simulink model "task_1_2_v01_2017b_compatible"  (R2018a)
settings: Solver=VariableStepAuto  StartTime=0.0  StopTime=1000  RelTol=1e-3
values from neighbouring files (symbols this model uses):
  faultMag = [1 0 0]    [ProblemData.m]
  faultTime = [1e6 1e6 1e6]    [ProblemData.m]
  lambda = 0.5    [ProblemData.m]
  pipeCoeff = [1 1 1]    [ProblemData.m]
  pipeCoeffNom = pipeCoeff * (1 + 0.1 * (rand(1) - 1/2))    [ProblemData.m]
  pipeCross = [5 5 5]*1e-4    [ProblemData.m]
  pipeCrossNom = pipeCross * (1 + 0.1 * (rand(1) - 1/2))    [ProblemData.m]
  pumpConst = [1.5 1.5]*1e-3    [ProblemData.m]
  seed1 = randi([1 100000])    [ProblemData.m]
  seed2 = randi([1 100000])    [ProblemData.m]
  seed3 = randi([1 100000])    [ProblemData.m]
  tankCross = [0.156 0.156 0.156]    [ProblemData.m]
  tankCrossNom = tankCross * (1 + 0.1 * (rand(1) - 1/2))    [ProblemData.m]
  tankInit = [0 2.5 5]    [ProblemData.m]
  tankInitNom = tankInit * (1 + 0.1 * (rand(1) - 1/2))    [ProblemData.m]
  tankMax = [10 10 10]    [ProblemData.m]
  tankMaxNom = tankMax * (1 + 0.1 * (rand(1) - 1/2))    [ProblemData.m]
  tankMin = [0 0 0]    [ProblemData.m]
undefined symbols (not defined in the file or in its folder): DiscIntNeverNeededParam
(part 1 of 2)
settings Model: Creator=riccardoferrar  LastModifiedBy=Casper

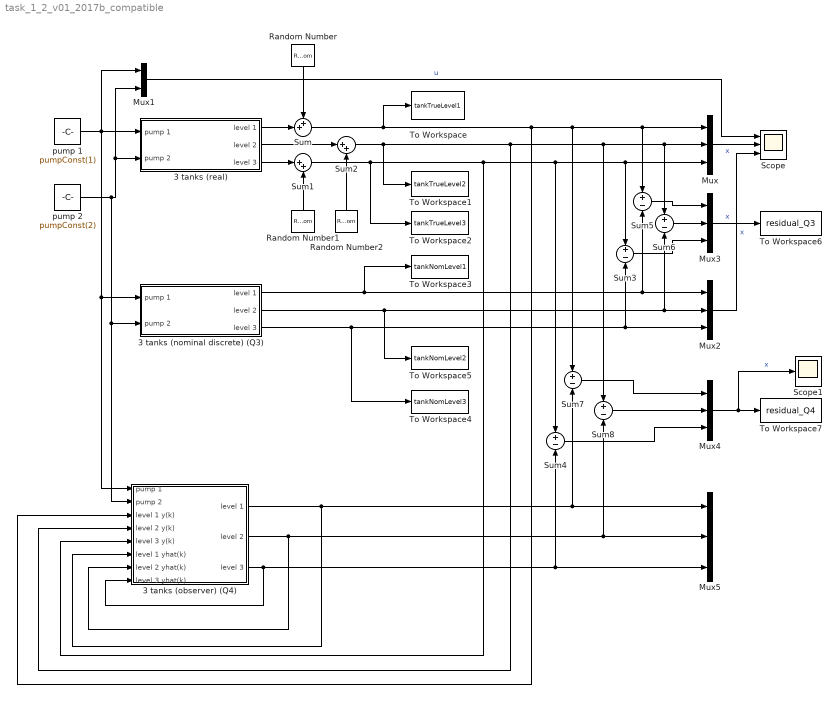
== system task_1_2_v01_2017b_compatible ==
  3 tanks (nominal discrete) (Q3) : Subsystem
  3 tanks (observer) (Q4) : Subsystem
  3 tanks (real) : Subsystem
  Mux{,2..5} (5 alike) : Mux  Inputs=3
  Mux1 : Mux  Inputs=2
  Random Number : RandomNumber  Variance=0.0015  Seed=seed1  SampleTime=0.1
  Random Number1 : RandomNumber  Variance=0.0015  Seed=seed2  SampleTime=0.1
  Random Number2 : RandomNumber  Variance=0.0015  Seed=seed3  SampleTime=0.1
  Scope : Scope  NumInputPorts=3
  Scope1 : Scope
  Sum : Sum  Inputs=++|
  Sum1 : Sum  Inputs=|++
  Sum2 : Sum  Inputs=|++
  Sum{3..8} (6 alike) : Sum  Inputs=+|-
  To Workspace : ToWorkspace  VariableName=tankTrueLevel1  SaveFormat=Timeseries  SampleTime=-1
  To Workspace1 : ToWorkspace  VariableName=tankTrueLevel2  SaveFormat=Timeseries  SampleTime=-1
  To Workspace2 : ToWorkspace  VariableName=tankTrueLevel3  SaveFormat=Timeseries  SampleTime=-1
  To Workspace3 : ToWorkspace  VariableName=tankNomLevel1  SaveFormat=Timeseries  SampleTime=-1
  To Workspace4 : ToWorkspace  VariableName=tankNomLevel3  SaveFormat=Timeseries  SampleTime=-1
  To Workspace5 : ToWorkspace  VariableName=tankNomLevel2  SaveFormat=Timeseries  SampleTime=-1
  To Workspace6 : ToWorkspace  VariableName=residual_Q3  SaveFormat=Timeseries  SampleTime=-1
  To Workspace7 : ToWorkspace  VariableName=residual_Q4  SaveFormat=Timeseries  SampleTime=-1
  pump 1 : Constant  Value=pumpConst(1)
  pump 2 : Constant  Value=pumpConst(2)
  wires:
  pump 1/1 -> 3 tanks (observer) (Q4)/1(pump 1), 3 tanks (nominal discrete) (Q3)/1(pump 1), 3 tanks (real)/1(pump 1), Mux1/1
  pump 2/1 -> 3 tanks (observer) (Q4)/2(pump 2), 3 tanks (nominal discrete) (Q3)/2(pump 2), Mux1/2, 3 tanks (real)/2(pump 2)
  Mux/1 -> Scope/2  "x"
  3 tanks (real)/1(level 1) -> Sum/2
  Random Number/1 -> Sum/1
  Sum/1 -> To Workspace/1, Sum7/1, Sum5/1, Mux/1, 3 tanks (observer) (Q4)/3(level 1 y(k))
  3 tanks (real)/2(level 2) -> Sum2/1
  Sum2/1 -> To Workspace1/1, Sum6/1, Mux/2, Sum8/1, 3 tanks (observer) (Q4)/4(level 2 y(k))
  Random Number2/1 -> Sum2/2
  3 tanks (real)/3(level 3) -> Sum1/1
  Random Number1/1 -> Sum1/2
  Sum1/1 -> To Workspace2/1, Sum3/1, Mux/3, Sum4/1, 3 tanks (observer) (Q4)/5(level 3 y(k))
  Mux1/1 -> Scope/1  "u"
  Mux2/1 -> Scope/3  "x"
  3 tanks (nominal discrete) (Q3)/1(level 1) -> To Workspace3/1, Sum5/2, Mux2/1
  3 tanks (nominal discrete) (Q3)/2(level 2) -> To Workspace5/1, Sum6/2, Mux2/2
  3 tanks (nominal discrete) (Q3)/3(level 3) -> To Workspace4/1, Sum3/2, Mux2/3
  Sum5/1 -> Mux3/1
  Sum6/1 -> Mux3/2
  Sum3/1 -> Mux3/3
  Mux3/1 -> To Workspace6/1  "x"
  Sum7/1 -> Mux4/1
  Mux4/1 -> Scope1/1, To Workspace7/1  "x"
  3 tanks (observer) (Q4)/1(level 1) -> 3 tanks (observer) (Q4)/6(level 1 yhat(k)), Sum7/2, Mux5/1
  3 tanks (observer) (Q4)/2(level 2) -> 3 tanks (observer) (Q4)/7(level 2 yhat(k)), Sum8/2, Mux5/2
  3 tanks (observer) (Q4)/3(level 3) -> Sum4/2, Mux5/3, 3 tanks (observer) (Q4)/8(level 3 yhat(k))
  Sum8/1 -> Mux4/2
  Sum4/1 -> Mux4/3

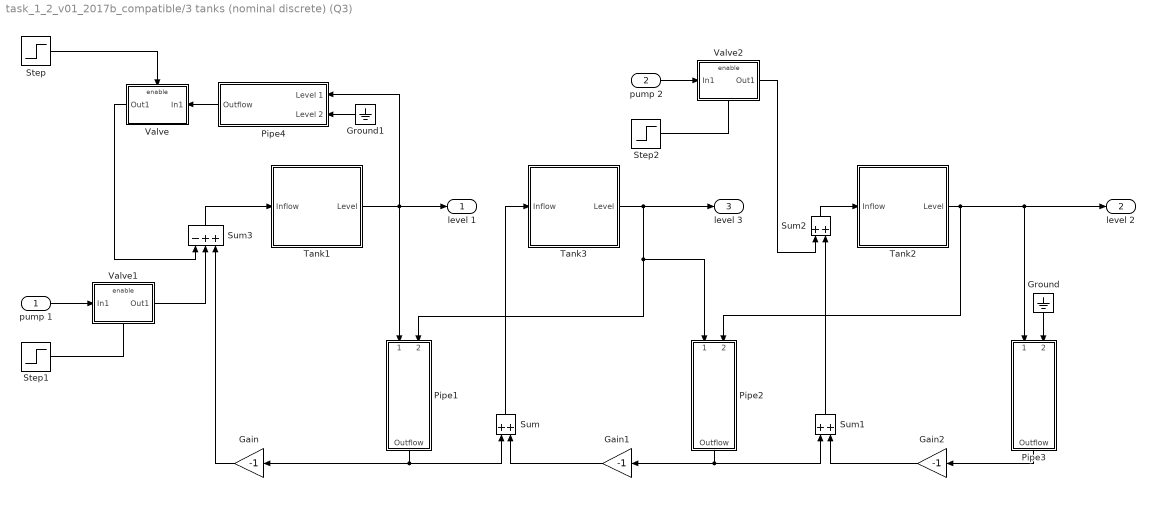
== system task_1_2_v01_2017b_compatible/3 tanks (nominal discrete) (Q3) ==
  pump 1 : Inport
  pump 2 : Inport  Port=2
  Gain : Gain  Gain=-1
  Gain1 : Gain  Gain=-1
  Gain2 : Gain  Gain=-1
  Ground : Ground
  Ground1 : Ground
  Pipe1 : Subsystem  mask(Connection Pipe){S_p=pipeCrossNom(1), c_o=pipeCoeffNom(1)}
      mask prompts: S_p "Pipe cross-section [m^2]"; c_o "Outflow coefficient"
      mask help:
      | Connection pipe between two tanks.
      | The pipe cross-section and the outflow coefficient are mask block parameters.
      mask Help:
      | Enter the pipe cross-section [S_p] and the outflow coefficient [c_o] in the block dialog parameter fields.
      | 
      | The block generates the pipe's flow-rate. The input signals are the level of fluid into both the tanks, connected by the pipe. If the level in the first tank is bigger than the level in the second one, the fluid flow from the first to the second tank, else in the opposite way.
      mask Display: image(imread('pipe.jpg'));
  Pipe2 : Subsystem  mask(Connection Pipe){S_p=pipeCross(2), c_o=pipeCoeff(2)}
      mask prompts: S_p "Pipe cross-section [m^2]"; c_o "Outflow coefficient"
      mask help:
      | Connection pipe between two tanks.
      | The pipe cross-section and the outflow coefficient are mask block parameters.
      mask Help:
      | Enter the pipe cross-section [S_p] and the outflow coefficient [c_o] in the block dialog parameter fields.
      | 
      | The block generates the pipe's flow-rate. The input signals are the level of fluid into both the tanks, connected by the pipe. If the level in the first tank is bigger than the level in the second one, the fluid flow from the first to the second tank, else in the opposite way.
      mask Display: image(imread('pipe.jpg'));
  Pipe3 : Subsystem  mask(Connection Pipe){S_p=pipeCross(3), c_o=pipeCoeff(3)}
      mask prompts: S_p "Pipe cross-section [m^2]"; c_o "Outflow coefficient"
      mask help:
      | Connection pipe between two tanks.
      | The pipe cross-section and the outflow coefficient are mask block parameters.
      mask Help:
      | Enter the pipe cross-section [S_p] and the outflow coefficient [c_o] in the block dialog parameter fields.
      | 
      | The block generates the pipe's flow-rate. The input signals are the level of fluid into both the tanks, connected by the pipe. If the level in the first tank is bigger than the level in the second one, the fluid flow from the first to the second tank, else in the opposite way.
      mask Display: image(imread('pipe.jpg'));
  Pipe4 : Subsystem  mask(Connection Pipe){S_p=faultMag(2), c_o=1}
      mask prompts: S_p "Pipe cross-section [m^2]"; c_o "Outflow coefficient"
      mask help:
      | Connection pipe between two tanks.
      | The pipe cross-section and the outflow coefficient are mask block parameters.
      mask Help:
      | Enter the pipe cross-section [S_p] and the outflow coefficient [c_o] in the block dialog parameter fields.
      | 
      | The block generates the pipe's flow-rate. The input signals are the level of fluid into both the tanks, connected by the pipe. If the level in the first tank is bigger than the level in the second one, the fluid flow from the first to the second tank, else in the opposite way.
      mask Display: image(imread('pipe.jpg'));
  Step : Step  Time=faultTime(2)  SampleTime=0
  Step1 : Step  Time=faultTime(1)  Before=1  After=1-faultMag(1)  SampleTime=0
  Step2 : Step  Time=faultTime(3)  Before=1  After=1-faultMag(3)  SampleTime=0
  Sum : Sum
  Sum1 : Sum
  Sum2 : Sum
  Sum3 : Sum  Inputs=-++
  Tank1 : Subsystem  mask(Tank system){S=tankCrossNom(1), x_0=tankInitNom(1), max_level=tankMaxNom(1), min_level=tankMin(1)}
      mask prompts: S "Tank cross-section [m^2]"; x_0 "Initial fluid level [m"; max_level "Maximum fluid level [m]"; min_level "Minimum fluid level [m]"
      mask help:
      | Model of  a simple tank system. The input is a fluid flow-rate (may be positive or negative), the output is the fluid level in the tank.
      |
      | The tank cross-section, the initial, minimum and maximum fluid level are mask block parameters.
      mask Help:
      | Enter the tank cross-section, the initial, minimum, maximum fluid level in the block dialog parameter fields.
      | 
      | The block models a simple tank system. The input is the fluid flow-rate (positive or negative) that feeds the system; the output is the fluid level in the tank.
      mask Display: image(imread('tank.jpg'));
  Tank2 : Subsystem  mask(Tank system){S=tankCrossNom(2), x_0=tankInitNom(2), max_level=tankMaxNom(2), min_level=tankMin(2)}
      mask prompts: S "Tank cross-section [m^2]"; x_0 "Initial fluid level [m"; max_level "Maximum fluid level [m]"; min_level "Minimum fluid level [m]"
      mask help:
      | Model of  a simple tank system. The input is a fluid flow-rate (may be positive or negative), the output is the fluid level in the tank.
      |
      | The tank cross-section, the initial, minimum and maximum fluid level are mask block parameters.
      mask Help:
      | Enter the tank cross-section, the initial, minimum, maximum fluid level in the block dialog parameter fields.
      | 
      | The block models a simple tank system. The input is the fluid flow-rate (positive or negative) that feeds the system; the output is the fluid level in the tank.
      mask Display: image(imread('tank.jpg'));
  Tank3 : Subsystem  mask(Tank system){S=tankCrossNom(3), x_0=tankInitNom(3), max_level=tankMaxNom(3), min_level=tankMin(3)}
      mask prompts: S "Tank cross-section [m^2]"; x_0 "Initial fluid level [m"; max_level "Maximum fluid level [m]"; min_level "Minimum fluid level [m]"
      mask help:
      | Model of  a simple tank system. The input is a fluid flow-rate (may be positive or negative), the output is the fluid level in the tank.
      |
      | The tank cross-section, the initial, minimum and maximum fluid level are mask block parameters.
      mask Help:
      | Enter the tank cross-section, the initial, minimum, maximum fluid level in the block dialog parameter fields.
      | 
      | The block models a simple tank system. The input is the fluid flow-rate (positive or negative) that feeds the system; the output is the fluid level in the tank.
      mask Display: image(imread('tank.jpg'));
  Valve : Subsystem  TreatAsAtomicUnit=on  mask(Valve subsystem){}
      mask help: Model of a valve. When the control signal is greather then 0, the output is equal to the input. Otherwise, the output is 0.
      mask Display: image(imread('valve.jpg'))
  Valve1 : Subsystem  TreatAsAtomicUnit=on  mask(Valve subsystem){}
      mask help: Model of a valve. When the control signal is greather then 0, the output is equal to the input. Otherwise, the output is 0.
      mask Display: image(imread('valve.jpg'))
  Valve2 : Subsystem  TreatAsAtomicUnit=on  mask(Valve subsystem){}
      mask help: Model of a valve. When the control signal is greather then 0, the output is equal to the input. Otherwise, the output is 0.
      mask Display: image(imread('valve.jpg'))
  level 1 : Outport
  level 2 : Outport  Port=2
  level 3 : Outport  Port=3
  wires:
  Sum/1 -> Tank3/1(Inflow)
  Gain1/1 -> Sum/2
  Pipe2/1(Outflow) -> Sum1/1, Gain1/1
  Gain/1 -> Sum3/3
  Tank2/1(Level) -> level 2/1, Pipe3/1(Level 1), Pipe2/2(Level 2)
  Sum1/1 -> Sum2/2
  Gain2/1 -> Sum1/2
  Pipe3/1(Outflow) -> Gain2/1
  Tank1/1(Level) -> Pipe4/1(Level 1), level 1/1, Pipe1/1(Level 1)
  Tank3/1(Level) -> level 3/1, Pipe2/1(Level 1), Pipe1/2(Level 2)
  Pipe1/1(Outflow) -> Sum/1, Gain/1
  Valve2/1(Out1) -> Sum2/1
  Sum2/1 -> Tank2/1(Inflow)
  Sum3/1 -> Tank1/1(Inflow)
  Ground/1 -> Pipe3/2(Level 2)
  Ground1/1 -> Pipe4/2(Level 2)
  Pipe4/1(Outflow) -> Valve/1(In1)
  Valve/1(Out1) -> Sum3/1
  Step/1 -> Valve/Enable
  pump 1/1 -> Valve1/1(In1)
  Valve1/1(Out1) -> Sum3/2
  Step1/1 -> Valve1/Enable
  Step2/1 -> Valve2/Enable
  pump 2/1 -> Valve2/1(In1)

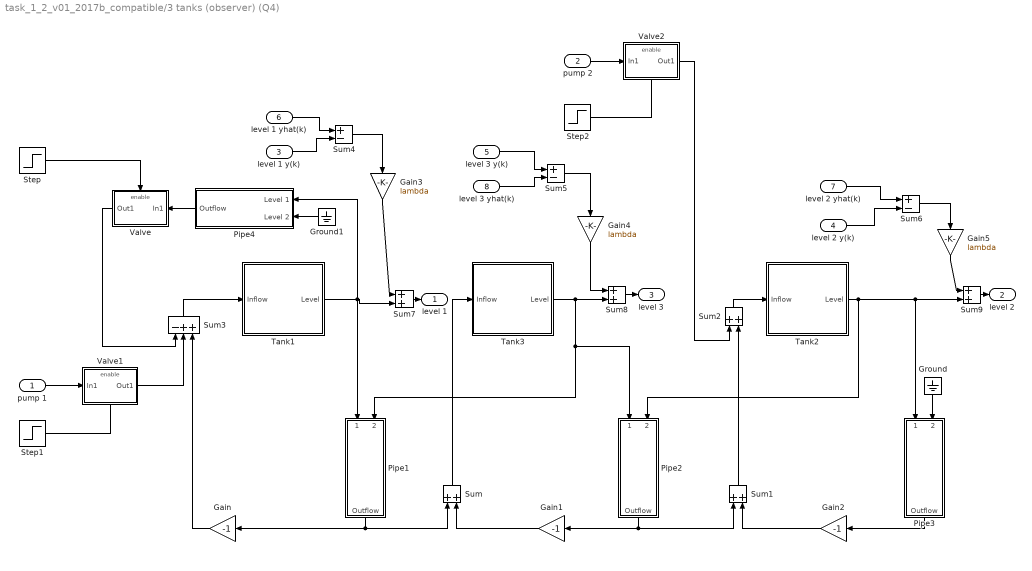
== system task_1_2_v01_2017b_compatible/3 tanks (observer) (Q4) ==
  pump 1 : Inport
  pump 2 : Inport  Port=2
  level 1 y(k) : Inport  Port=3
  level 2 y(k) : Inport  Port=4
  level 3 y(k) : Inport  Port=5
  level 1 yhat(k) : Inport  Port=6
  level 2 yhat(k) : Inport  Port=7
  level 3 yhat(k) : Inport  Port=8
  Gain : Gain  Gain=-1
  Gain1 : Gain  Gain=-1
  Gain2 : Gain  Gain=-1
  Gain3 : Gain  Gain=lambda
  Gain4 : Gain  Gain=lambda
  Gain5 : Gain  Gain=lambda
  Ground : Ground
  Ground1 : Ground
  Pipe1 : Subsystem  mask(Connection Pipe){S_p=pipeCrossNom(1), c_o=pipeCoeffNom(1)}
      mask prompts: S_p "Pipe cross-section [m^2]"; c_o "Outflow coefficient"
      mask help:
      | Connection pipe between two tanks.
      | The pipe cross-section and the outflow coefficient are mask block parameters.
      mask Help:
      | Enter the pipe cross-section [S_p] and the outflow coefficient [c_o] in the block dialog parameter fields.
      | 
      | The block generates the pipe's flow-rate. The input signals are the level of fluid into both the tanks, connected by the pipe. If the level in the first tank is bigger than the level in the second one, the fluid flow from the first to the second tank, else in the opposite way.
      mask Display: image(imread('pipe.jpg'));
  Pipe2 : Subsystem  mask(Connection Pipe){S_p=pipeCross(2), c_o=pipeCoeff(2)}
      mask prompts: S_p "Pipe cross-section [m^2]"; c_o "Outflow coefficient"
      mask help:
      | Connection pipe between two tanks.
      | The pipe cross-section and the outflow coefficient are mask block parameters.
      mask Help:
      | Enter the pipe cross-section [S_p] and the outflow coefficient [c_o] in the block dialog parameter fields.
      | 
      | The block generates the pipe's flow-rate. The input signals are the level of fluid into both the tanks, connected by the pipe. If the level in the first tank is bigger than the level in the second one, the fluid flow from the first to the second tank, else in the opposite way.
      mask Display: image(imread('pipe.jpg'));
  Pipe3 : Subsystem  mask(Connection Pipe){S_p=pipeCross(3), c_o=pipeCoeff(3)}
      mask prompts: S_p "Pipe cross-section [m^2]"; c_o "Outflow coefficient"
      mask help:
      | Connection pipe between two tanks.
      | The pipe cross-section and the outflow coefficient are mask block parameters.
      mask Help:
      | Enter the pipe cross-section [S_p] and the outflow coefficient [c_o] in the block dialog parameter fields.
      | 
      | The block generates the pipe's flow-rate. The input signals are the level of fluid into both the tanks, connected by the pipe. If the level in the first tank is bigger than the level in the second one, the fluid flow from the first to the second tank, else in the opposite way.
      mask Display: image(imread('pipe.jpg'));
  Pipe4 : Subsystem  mask(Connection Pipe){S_p=faultMag(2), c_o=1}
      mask prompts: S_p "Pipe cross-section [m^2]"; c_o "Outflow coefficient"
      mask help:
      | Connection pipe between two tanks.
      | The pipe cross-section and the outflow coefficient are mask block parameters.
      mask Help:
      | Enter the pipe cross-section [S_p] and the outflow coefficient [c_o] in the block dialog parameter fields.
      | 
      | The block generates the pipe's flow-rate. The input signals are the level of fluid into both the tanks, connected by the pipe. If the level in the first tank is bigger than the level in the second one, the fluid flow from the first to the second tank, else in the opposite way.
      mask Display: image(imread('pipe.jpg'));
  Step : Step  Time=faultTime(2)  SampleTime=0
  Step1 : Step  Time=faultTime(1)  Before=1  After=1-faultMag(1)  SampleTime=0
  Step2 : Step  Time=faultTime(3)  Before=1  After=1-faultMag(3)  SampleTime=0
  Sum{,1..2,7..9} (6 alike) : Sum
  Sum3 : Sum  Inputs=-++
  Sum4 : Sum  Inputs=+-
  Sum5 : Sum  Inputs=+-
  Sum6 : Sum  Inputs=+-
  Tank1 : Subsystem  mask(Tank system){S=tankCrossNom(1), x_0=tankInitNom(1), max_level=tankMaxNom(1), min_level=tankMin(1)}
      mask prompts: S "Tank cross-section [m^2]"; x_0 "Initial fluid level [m"; max_level "Maximum fluid level [m]"; min_level "Minimum fluid level [m]"
      mask help:
      | Model of  a simple tank system. The input is a fluid flow-rate (may be positive or negative), the output is the fluid level in the tank.
      |
      | The tank cross-section, the initial, minimum and maximum fluid level are mask block parameters.
      mask Help:
      | Enter the tank cross-section, the initial, minimum, maximum fluid level in the block dialog parameter fields.
      | 
      | The block models a simple tank system. The input is the fluid flow-rate (positive or negative) that feeds the system; the output is the fluid level in the tank.
      mask Display: image(imread('tank.jpg'));
  Tank2 : Subsystem  mask(Tank system){S=tankCrossNom(2), x_0=tankInitNom(2), max_level=tankMaxNom(2), min_level=tankMin(2)}
      mask prompts: S "Tank cross-section [m^2]"; x_0 "Initial fluid level [m"; max_level "Maximum fluid level [m]"; min_level "Minimum fluid level [m]"
      mask help:
      | Model of  a simple tank system. The input is a fluid flow-rate (may be positive or negative), the output is the fluid level in the tank.
      |
      | The tank cross-section, the initial, minimum and maximum fluid level are mask block parameters.
      mask Help:
      | Enter the tank cross-section, the initial, minimum, maximum fluid level in the block dialog parameter fields.
      | 
      | The block models a simple tank system. The input is the fluid flow-rate (positive or negative) that feeds the system; the output is the fluid level in the tank.
      mask Display: image(imread('tank.jpg'));
  Tank3 : Subsystem  mask(Tank system){S=tankCrossNom(3), x_0=tankInitNom(3), max_level=tankMaxNom(3), min_level=tankMin(3)}
      mask prompts: S "Tank cross-section [m^2]"; x_0 "Initial fluid level [m"; max_level "Maximum fluid level [m]"; min_level "Minimum fluid level [m]"
      mask help:
      | Model of  a simple tank system. The input is a fluid flow-rate (may be positive or negative), the output is the fluid level in the tank.
      |
      | The tank cross-section, the initial, minimum and maximum fluid level are mask block parameters.
      mask Help:
      | Enter the tank cross-section, the initial, minimum, maximum fluid level in the block dialog parameter fields.
      | 
      | The block models a simple tank system. The input is the fluid flow-rate (positive or negative) that feeds the system; the output is the fluid level in the tank.
      mask Display: image(imread('tank.jpg'));
  Valve : Subsystem  TreatAsAtomicUnit=on  mask(Valve subsystem){}
      mask help: Model of a valve. When the control signal is greather then 0, the output is equal to the input. Otherwise, the output is 0.
      mask Display: image(imread('valve.jpg'))
  Valve1 : Subsystem  TreatAsAtomicUnit=on  mask(Valve subsystem){}
      mask help: Model of a valve. When the control signal is greather then 0, the output is equal to the input. Otherwise, the output is 0.
      mask Display: image(imread('valve.jpg'))
  Valve2 : Subsystem  TreatAsAtomicUnit=on  mask(Valve subsystem){}
      mask help: Model of a valve. When the control signal is greather then 0, the output is equal to the input. Otherwise, the output is 0.
      mask Display: image(imread('valve.jpg'))
  level 1 : Outport
  level 2 : Outport  Port=2
  level 3 : Outport  Port=3
  wires:
  Sum/1 -> Tank3/1(Inflow)
  Gain1/1 -> Sum/2
  Pipe2/1(Outflow) -> Sum1/1, Gain1/1
  Gain/1 -> Sum3/3
  Tank2/1(Level) -> Sum9/2, Pipe3/1(Level 1), Pipe2/2(Level 2)
  Sum1/1 -> Sum2/2
  Gain2/1 -> Sum1/2
  Pipe3/1(Outflow) -> Gain2/1
  Tank1/1(Level) -> Sum7/2, Pipe4/1(Level 1), Pipe1/1(Level 1)
  Tank3/1(Level) -> Pipe2/1(Level 1), Pipe1/2(Level 2), Sum8/2
  Pipe1/1(Outflow) -> Sum/1, Gain/1
  Valve2/1(Out1) -> Sum2/1
  Sum2/1 -> Tank2/1(Inflow)
  Sum3/1 -> Tank1/1(Inflow)
  Ground/1 -> Pipe3/2(Level 2)
  Ground1/1 -> Pipe4/2(Level 2)
  Pipe4/1(Outflow) -> Valve/1(In1)
  Valve/1(Out1) -> Sum3/1
  Step/1 -> Valve/Enable
  pump 1/1 -> Valve1/1(In1)
  Valve1/1(Out1) -> Sum3/2
  Step1/1 -> Valve1/Enable
  Step2/1 -> Valve2/Enable
  pump 2/1 -> Valve2/1(In1)
  level 1 yhat(k)/1 -> Sum4/1
  level 1 y(k)/1 -> Sum4/2
  Sum7/1 -> level 1/1
  Sum4/1 -> Gain3/1
  Gain3/1 -> Sum7/1
  level 3 y(k)/1 -> Sum5/1
  level 3 yhat(k)/1 -> Sum5/2
  Sum5/1 -> Gain4/1
  Sum8/1 -> level 3/1
  Gain4/1 -> Sum8/1
  level 2 yhat(k)/1 -> Sum6/1
  level 2 y(k)/1 -> Sum6/2
  Sum6/1 -> Gain5/1
  Sum9/1 -> level 2/1
  Gain5/1 -> Sum9/1

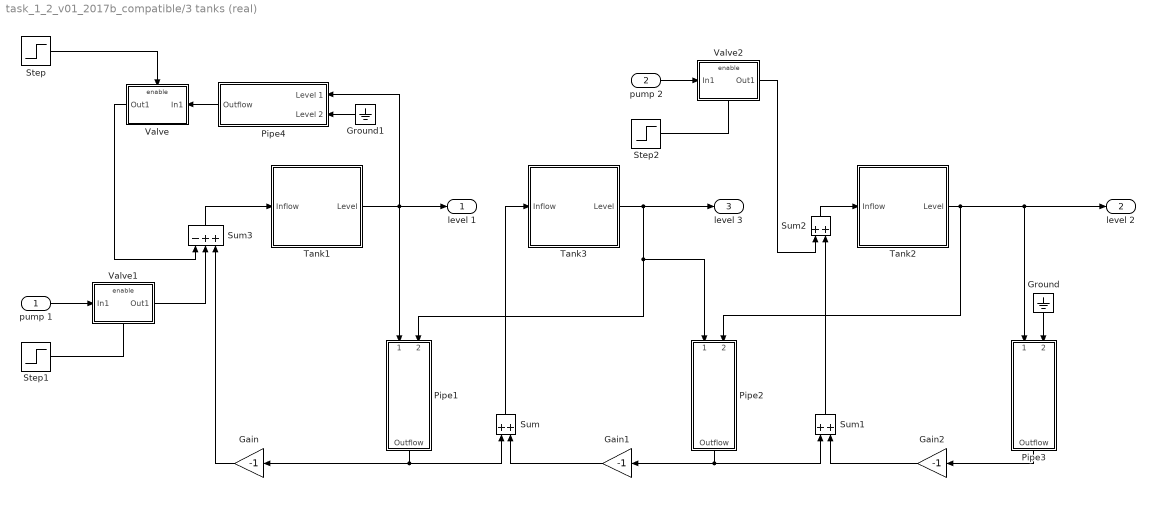
== system task_1_2_v01_2017b_compatible/3 tanks (real) ==
  pump 1 : Inport
  pump 2 : Inport  Port=2
  Gain : Gain  Gain=-1
  Gain1 : Gain  Gain=-1
  Gain2 : Gain  Gain=-1
  Ground : Ground
  Ground1 : Ground
  Pipe1 : Subsystem  mask(Connection Pipe){S_p=pipeCross(1), c_o=pipeCoeff(1)}
      mask prompts: S_p "Pipe cross-section [m^2]"; c_o "Outflow coefficient"
      mask help:
      | Connection pipe between two tanks.
      | The pipe cross-section and the outflow coefficient are mask block parameters.
      mask Help:
      | Enter the pipe cross-section [S_p] and the outflow coefficient [c_o] in the block dialog parameter fields.
      | 
      | The block generates the pipe's flow-rate. The input signals are the level of fluid into both the tanks, connected by the pipe. If the level in the first tank is bigger than the level in the second one, the fluid flow from the first to the second tank, else in the opposite way.
      mask Display: image(imread('pipe.jpg'));
  Pipe2 : Subsystem  mask(Connection Pipe){S_p=pipeCross(2), c_o=pipeCoeff(2)}
      mask prompts: S_p "Pipe cross-section [m^2]"; c_o "Outflow coefficient"
      mask help:
      | Connection pipe between two tanks.
      | The pipe cross-section and the outflow coefficient are mask block parameters.
      mask Help:
      | Enter the pipe cross-section [S_p] and the outflow coefficient [c_o] in the block dialog parameter fields.
      | 
      | The block generates the pipe's flow-rate. The input signals are the level of fluid into both the tanks, connected by the pipe. If the level in the first tank is bigger than the level in the second one, the fluid flow from the first to the second tank, else in the opposite way.
      mask Display: image(imread('pipe.jpg'));
  Pipe3 : Subsystem  mask(Connection Pipe){S_p=pipeCross(3), c_o=pipeCoeff(3)}
      mask prompts: S_p "Pipe cross-section [m^2]"; c_o "Outflow coefficient"
      mask help:
      | Connection pipe between two tanks.
      | The pipe cross-section and the outflow coefficient are mask block parameters.
      mask Help:
      | Enter the pipe cross-section [S_p] and the outflow coefficient [c_o] in the block dialog parameter fields.
      | 
      | The block generates the pipe's flow-rate. The input signals are the level of fluid into both the tanks, connected by the pipe. If the level in the first tank is bigger than the level in the second one, the fluid flow from the first to the second tank, else in the opposite way.
      mask Display: image(imread('pipe.jpg'));
  Pipe4 : Subsystem  mask(Connection Pipe){S_p=faultMag(2), c_o=1}
      mask prompts: S_p "Pipe cross-section [m^2]"; c_o "Outflow coefficient"
      mask help:
      | Connection pipe between two tanks.
      | The pipe cross-section and the outflow coefficient are mask block parameters.
      mask Help:
      | Enter the pipe cross-section [S_p] and the outflow coefficient [c_o] in the block dialog parameter fields.
      | 
      | The block generates the pipe's flow-rate. The input signals are the level of fluid into both the tanks, connected by the pipe. If the level in the first tank is bigger than the level in the second one, the fluid flow from the first to the second tank, else in the opposite way.
      mask Display: image(imread('pipe.jpg'));
  Step : Step  Time=faultTime(2)  SampleTime=0
  Step1 : Step  Time=faultTime(1)  Before=1  After=1-faultMag(1)  SampleTime=0
  Step2 : Step  Time=faultTime(3)  Before=1  After=1-faultMag(3)  SampleTime=0
  Sum : Sum
  Sum1 : Sum
  Sum2 : Sum
  Sum3 : Sum  Inputs=-++
  Tank1 : Subsystem  mask(Tank system){S=tankCross(1), x_0=tankInit(1), max_level=tankMax(1), min_level=tankMin(1)}
      mask prompts: S "Tank cross-section [m^2]"; x_0 "Initial fluid level [m"; max_level "Maximum fluid level [m]"; min_level "Minimum fluid level [m]"
      mask help:
      | Model of  a simple tank system. The input is a fluid flow-rate (may be positive or negative), the output is the fluid level in the tank.
      |
      | The tank cross-section, the initial, minimum and maximum fluid level are mask block parameters.
      mask Help:
      | Enter the tank cross-section, the initial, minimum, maximum fluid level in the block dialog parameter fields.
      | 
      | The block models a simple tank system. The input is the fluid flow-rate (positive or negative) that feeds the system; the output is the fluid level in the tank.
      mask Display: image(imread('tank.jpg'));
  Tank2 : Subsystem  mask(Tank system){S=tankCross(2), x_0=tankInit(2), max_level=tankMax(2), min_level=tankMin(2)}
      mask prompts: S "Tank cross-section [m^2]"; x_0 "Initial fluid level [m"; max_level "Maximum fluid level [m]"; min_level "Minimum fluid level [m]"
      mask help:
      | Model of  a simple tank system. The input is a fluid flow-rate (may be positive or negative), the output is the fluid level in the tank.
      |
      | The tank cross-section, the initial, minimum and maximum fluid level are mask block parameters.
      mask Help:
      | Enter the tank cross-section, the initial, minimum, maximum fluid level in the block dialog parameter fields.
      | 
      | The block models a simple tank system. The input is the fluid flow-rate (positive or negative) that feeds the system; the output is the fluid level in the tank.
      mask Display: image(imread('tank.jpg'));
  Tank3 : Subsystem  mask(Tank system){S=tankCross(3), x_0=tankInit(3), max_level=tankMax(3), min_level=tankMin(3)}
      mask prompts: S "Tank cross-section [m^2]"; x_0 "Initial fluid level [m"; max_level "Maximum fluid level [m]"; min_level "Minimum fluid level [m]"
      mask help:
      | Model of  a simple tank system. The input is a fluid flow-rate (may be positive or negative), the output is the fluid level in the tank.
      |
      | The tank cross-section, the initial, minimum and maximum fluid level are mask block parameters.
      mask Help:
      | Enter the tank cross-section, the initial, minimum, maximum fluid level in the block dialog parameter fields.
      | 
      | The block models a simple tank system. The input is the fluid flow-rate (positive or negative) that feeds the system; the output is the fluid level in the tank.
      mask Display: image(imread('tank.jpg'));
  Valve : Subsystem  TreatAsAtomicUnit=on  mask(Valve subsystem){}
      mask help: Model of a valve. When the control signal is greather then 0, the output is equal to the input. Otherwise, the output is 0.
      mask Display: image(imread('valve.jpg'))
  Valve1 : Subsystem  TreatAsAtomicUnit=on  mask(Valve subsystem){}
      mask help: Model of a valve. When the control signal is greather then 0, the output is equal to the input. Otherwise, the output is 0.
      mask Display: image(imread('valve.jpg'))
  Valve2 : Subsystem  TreatAsAtomicUnit=on  mask(Valve subsystem){}
      mask help: Model of a valve. When the control signal is greather then 0, the output is equal to the input. Otherwise, the output is 0.
      mask Display: image(imread('valve.jpg'))
  level 1 : Outport
  level 2 : Outport  Port=2
  level 3 : Outport  Port=3
  wires:
  Sum/1 -> Tank3/1(Inflow)
  Gain1/1 -> Sum/2
  Pipe2/1(Outflow) -> Sum1/1, Gain1/1
  Gain/1 -> Sum3/3
  Tank2/1(Level) -> level 2/1, Pipe3/1(Level 1), Pipe2/2(Level 2)
  Sum1/1 -> Sum2/2
  Gain2/1 -> Sum1/2
  Pipe3/1(Outflow) -> Gain2/1
  Tank1/1(Level) -> Pipe4/1(Level 1), level 1/1, Pipe1/1(Level 1)
  Tank3/1(Level) -> level 3/1, Pipe2/1(Level 1), Pipe1/2(Level 2)
  Pipe1/1(Outflow) -> Sum/1, Gain/1
  Valve2/1(Out1) -> Sum2/1
  Sum2/1 -> Tank2/1(Inflow)
  Sum3/1 -> Tank1/1(Inflow)
  Ground/1 -> Pipe3/2(Level 2)
  Ground1/1 -> Pipe4/2(Level 2)
  Pipe4/1(Outflow) -> Valve/1(In1)
  Valve/1(Out1) -> Sum3/1
  Step/1 -> Valve/Enable
  pump 1/1 -> Valve1/1(In1)
  Valve1/1(Out1) -> Sum3/2
  Step1/1 -> Valve1/Enable
  Step2/1 -> Valve2/Enable
  pump 2/1 -> Valve2/1(In1)

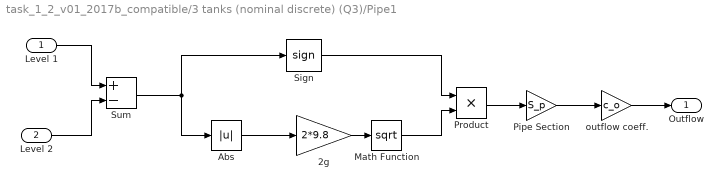
== system task_1_2_v01_2017b_compatible/3 tanks (nominal discrete) (Q3)/Pipe1 ==
  Level 1 : Inport
  Level 2 : Inport  Port=2
  2g : Gain  Gain=2*9.8  SaturateOnIntegerOverflow=on  OutDataTypeStr=Inherit: Same as input  ParamDataTypeStr=Inherit: Same as input
  Abs : Abs  SaturateOnIntegerOverflow=on
  Math Function : Math  Operator=sqrt  SaturateOnIntegerOverflow=on
  Pipe Section : Gain  Gain=S_p  SaturateOnIntegerOverflow=on  OutDataTypeStr=Inherit: Same as input  ParamDataTypeStr=Inherit: Same as input
  Product : Product  SaturateOnIntegerOverflow=on  InputSameDT=on  OutDataTypeStr=Inherit: Same as first input
  Sign : Signum
  Sum : Sum  Inputs=+-  SaturateOnIntegerOverflow=on  InputSameDT=on  OutDataTypeStr=Inherit: Same as first input
  outflow coeff. : Gain  Gain=c_o  SaturateOnIntegerOverflow=on  OutDataTypeStr=Inherit: Same as input  ParamDataTypeStr=Inherit: Same as input
  Outflow : Outport
  wires:
  outflow coeff./1 -> Outflow/1
  Pipe Section/1 -> outflow coeff./1
  Product/1 -> Pipe Section/1
  Sign/1 -> Product/1
  Math Function/1 -> Product/2
  2g/1 -> Math Function/1
  Abs/1 -> 2g/1
  Sum/1 -> Abs/1, Sign/1
  Level 2/1 -> Sum/2
  Level 1/1 -> Sum/1

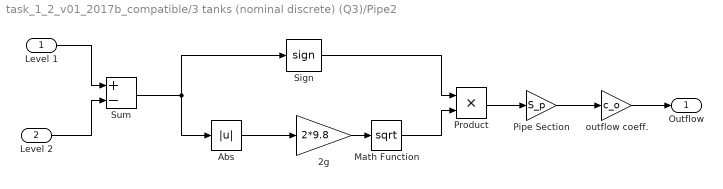
== system task_1_2_v01_2017b_compatible/3 tanks (nominal discrete) (Q3)/Pipe2 ==
  Level 1 : Inport
  Level 2 : Inport  Port=2
  2g : Gain  Gain=2*9.8  SaturateOnIntegerOverflow=on  OutDataTypeStr=Inherit: Same as input  ParamDataTypeStr=Inherit: Same as input
  Abs : Abs  SaturateOnIntegerOverflow=on
  Math Function : Math  Operator=sqrt  SaturateOnIntegerOverflow=on
  Pipe Section : Gain  Gain=S_p  SaturateOnIntegerOverflow=on  OutDataTypeStr=Inherit: Same as input  ParamDataTypeStr=Inherit: Same as input
  Product : Product  SaturateOnIntegerOverflow=on  InputSameDT=on  OutDataTypeStr=Inherit: Same as first input
  Sign : Signum
  Sum : Sum  Inputs=+-  SaturateOnIntegerOverflow=on  InputSameDT=on  OutDataTypeStr=Inherit: Same as first input
  outflow coeff. : Gain  Gain=c_o  SaturateOnIntegerOverflow=on  OutDataTypeStr=Inherit: Same as input  ParamDataTypeStr=Inherit: Same as input
  Outflow : Outport
  wires:
  outflow coeff./1 -> Outflow/1
  Pipe Section/1 -> outflow coeff./1
  Product/1 -> Pipe Section/1
  Sign/1 -> Product/1
  Math Function/1 -> Product/2
  2g/1 -> Math Function/1
  Abs/1 -> 2g/1
  Sum/1 -> Abs/1, Sign/1
  Level 2/1 -> Sum/2
  Level 1/1 -> Sum/1

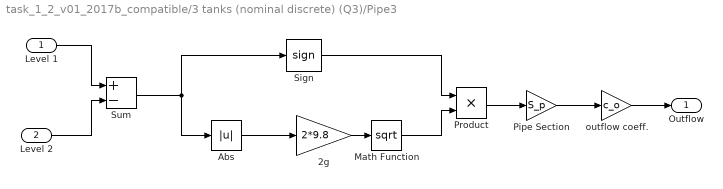
== system task_1_2_v01_2017b_compatible/3 tanks (nominal discrete) (Q3)/Pipe3 ==
  Level 1 : Inport
  Level 2 : Inport  Port=2
  2g : Gain  Gain=2*9.8  SaturateOnIntegerOverflow=on  OutDataTypeStr=Inherit: Same as input  ParamDataTypeStr=Inherit: Same as input
  Abs : Abs  SaturateOnIntegerOverflow=on
  Math Function : Math  Operator=sqrt  SaturateOnIntegerOverflow=on
  Pipe Section : Gain  Gain=S_p  SaturateOnIntegerOverflow=on  OutDataTypeStr=Inherit: Same as input  ParamDataTypeStr=Inherit: Same as input
  Product : Product  SaturateOnIntegerOverflow=on  InputSameDT=on  OutDataTypeStr=Inherit: Same as first input
  Sign : Signum
  Sum : Sum  Inputs=+-  SaturateOnIntegerOverflow=on  InputSameDT=on  OutDataTypeStr=Inherit: Same as first input
  outflow coeff. : Gain  Gain=c_o  SaturateOnIntegerOverflow=on  OutDataTypeStr=Inherit: Same as input  ParamDataTypeStr=Inherit: Same as input
  Outflow : Outport
  wires:
  outflow coeff./1 -> Outflow/1
  Pipe Section/1 -> outflow coeff./1
  Product/1 -> Pipe Section/1
  Sign/1 -> Product/1
  Math Function/1 -> Product/2
  2g/1 -> Math Function/1
  Abs/1 -> 2g/1
  Sum/1 -> Abs/1, Sign/1
  Level 2/1 -> Sum/2
  Level 1/1 -> Sum/1

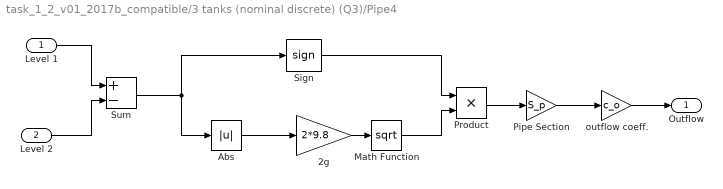
== system task_1_2_v01_2017b_compatible/3 tanks (nominal discrete) (Q3)/Pipe4 ==
  Level 1 : Inport
  Level 2 : Inport  Port=2
  2g : Gain  Gain=2*9.8  SaturateOnIntegerOverflow=on  OutDataTypeStr=Inherit: Same as input  ParamDataTypeStr=Inherit: Same as input
  Abs : Abs  SaturateOnIntegerOverflow=on
  Math Function : Math  Operator=sqrt  SaturateOnIntegerOverflow=on
  Pipe Section : Gain  Gain=S_p  SaturateOnIntegerOverflow=on  OutDataTypeStr=Inherit: Same as input  ParamDataTypeStr=Inherit: Same as input
  Product : Product  SaturateOnIntegerOverflow=on  InputSameDT=on  OutDataTypeStr=Inherit: Same as first input
  Sign : Signum
  Sum : Sum  Inputs=+-  SaturateOnIntegerOverflow=on  InputSameDT=on  OutDataTypeStr=Inherit: Same as first input
  outflow coeff. : Gain  Gain=c_o  SaturateOnIntegerOverflow=on  OutDataTypeStr=Inherit: Same as input  ParamDataTypeStr=Inherit: Same as input
  Outflow : Outport
  wires:
  outflow coeff./1 -> Outflow/1
  Pipe Section/1 -> outflow coeff./1
  Product/1 -> Pipe Section/1
  Sign/1 -> Product/1
  Math Function/1 -> Product/2
  2g/1 -> Math Function/1
  Abs/1 -> 2g/1
  Sum/1 -> Abs/1, Sign/1
  Level 2/1 -> Sum/2
  Level 1/1 -> Sum/1

== system task_1_2_v01_2017b_compatible/3 tanks (nominal discrete) (Q3)/Tank1 ==
  Inflow : Inport
  Discrete-Time Integrator : DiscreteIntegrator  InitialCondition=x_0  SampleTime=-1  OutMin=min_level  OutMax=max_level  ICPrevOutput=DiscIntNeverNeededParam  ICPrevScaledInput=DiscIntNeverNeededParam
  Tank Section : Gain  Gain=1/S  SaturateOnIntegerOverflow=on  OutDataTypeStr=Inherit: Same as input  ParamDataTypeStr=Inherit: Same as input
  Level : Outport  InitialOutput=0
  wires:
  Discrete-Time Integrator/1 -> Level/1
  Tank Section/1 -> Discrete-Time Integrator/1
  Inflow/1 -> Tank Section/1

== system task_1_2_v01_2017b_compatible/3 tanks (nominal discrete) (Q3)/Tank2 ==
  Inflow : Inport
  Discrete-Time Integrator : DiscreteIntegrator  InitialCondition=x_0  SampleTime=-1  OutMin=min_level  OutMax=max_level  ICPrevOutput=DiscIntNeverNeededParam  ICPrevScaledInput=DiscIntNeverNeededParam
  Tank Section : Gain  Gain=1/S  SaturateOnIntegerOverflow=on  OutDataTypeStr=Inherit: Same as input  ParamDataTypeStr=Inherit: Same as input
  Level : Outport  InitialOutput=0
  wires:
  Inflow/1 -> Tank Section/1
  Discrete-Time Integrator/1 -> Level/1
  Tank Section/1 -> Discrete-Time Integrator/1

== system task_1_2_v01_2017b_compatible/3 tanks (nominal discrete) (Q3)/Tank3 ==
  Inflow : Inport
  Discrete-Time Integrator : DiscreteIntegrator  InitialCondition=x_0  SampleTime=-1  OutMin=min_level  OutMax=max_level  ICPrevOutput=DiscIntNeverNeededParam  ICPrevScaledInput=DiscIntNeverNeededParam
  Tank Section : Gain  Gain=1/S  SaturateOnIntegerOverflow=on  OutDataTypeStr=Inherit: Same as input  ParamDataTypeStr=Inherit: Same as input
  Level : Outport  InitialOutput=0
  wires:
  Discrete-Time Integrator/1 -> Level/1
  Inflow/1 -> Tank Section/1
  Tank Section/1 -> Discrete-Time Integrator/1

== system task_1_2_v01_2017b_compatible/3 tanks (nominal discrete) (Q3)/Valve ==
  In1 : Inport
  Enable : EnablePort  StatesWhenEnabling=reset  ShowOutputPort=on
  Product : Product  SaturateOnIntegerOverflow=on  InputSameDT=on  OutDataTypeStr=Inherit: Same as first input
  Saturation : Saturate  UpperLimit=1.0  LowerLimit=0.0
  Out1 : Outport  OutputWhenDisabled=reset  InitialOutput=0
  wires:
  Enable/1 -> Saturation/1
  Saturation/1 -> Product/1
  In1/1 -> Product/2
  Product/1 -> Out1/1

== system task_1_2_v01_2017b_compatible/3 tanks (nominal discrete) (Q3)/Valve1 ==
  In1 : Inport
  Enable : EnablePort  StatesWhenEnabling=reset  ShowOutputPort=on
  Product : Product  SaturateOnIntegerOverflow=on  InputSameDT=on  OutDataTypeStr=Inherit: Same as first input
  Saturation : Saturate  UpperLimit=1.0  LowerLimit=0.0
  Out1 : Outport  OutputWhenDisabled=reset  InitialOutput=0
  wires:
  Enable/1 -> Saturation/1
  Saturation/1 -> Product/1
  In1/1 -> Product/2
  Product/1 -> Out1/1

== system task_1_2_v01_2017b_compatible/3 tanks (nominal discrete) (Q3)/Valve2 ==
  In1 : Inport
  Enable : EnablePort  StatesWhenEnabling=reset  ShowOutputPort=on
  Product : Product  SaturateOnIntegerOverflow=on  InputSameDT=on  OutDataTypeStr=Inherit: Same as first input
  Saturation : Saturate  UpperLimit=1.0  LowerLimit=0.0
  Out1 : Outport  OutputWhenDisabled=reset  InitialOutput=0
  wires:
  Enable/1 -> Saturation/1
  Saturation/1 -> Product/1
  In1/1 -> Product/2
  Product/1 -> Out1/1

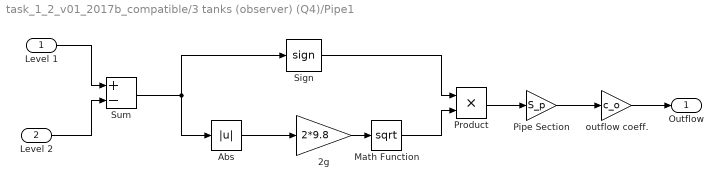
== system task_1_2_v01_2017b_compatible/3 tanks (observer) (Q4)/Pipe1 ==
  Level 1 : Inport
  Level 2 : Inport  Port=2
  2g : Gain  Gain=2*9.8  SaturateOnIntegerOverflow=on  OutDataTypeStr=Inherit: Same as input  ParamDataTypeStr=Inherit: Same as input
  Abs : Abs  SaturateOnIntegerOverflow=on
  Math Function : Math  Operator=sqrt  SaturateOnIntegerOverflow=on
  Pipe Section : Gain  Gain=S_p  SaturateOnIntegerOverflow=on  OutDataTypeStr=Inherit: Same as input  ParamDataTypeStr=Inherit: Same as input
  Product : Product  SaturateOnIntegerOverflow=on  InputSameDT=on  OutDataTypeStr=Inherit: Same as first input
  Sign : Signum
  Sum : Sum  Inputs=+-  SaturateOnIntegerOverflow=on  InputSameDT=on  OutDataTypeStr=Inherit: Same as first input
  outflow coeff. : Gain  Gain=c_o  SaturateOnIntegerOverflow=on  OutDataTypeStr=Inherit: Same as input  ParamDataTypeStr=Inherit: Same as input
  Outflow : Outport
  wires:
  outflow coeff./1 -> Outflow/1
  Pipe Section/1 -> outflow coeff./1
  Product/1 -> Pipe Section/1
  Sign/1 -> Product/1
  Math Function/1 -> Product/2
  2g/1 -> Math Function/1
  Abs/1 -> 2g/1
  Sum/1 -> Abs/1, Sign/1
  Level 2/1 -> Sum/2
  Level 1/1 -> Sum/1

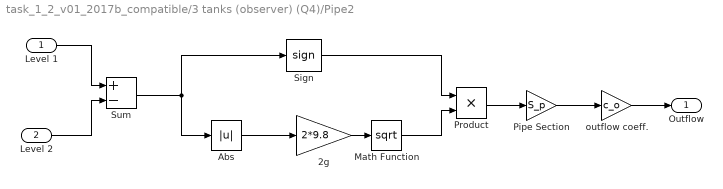
== system task_1_2_v01_2017b_compatible/3 tanks (observer) (Q4)/Pipe2 ==
  Level 1 : Inport
  Level 2 : Inport  Port=2
  2g : Gain  Gain=2*9.8  SaturateOnIntegerOverflow=on  OutDataTypeStr=Inherit: Same as input  ParamDataTypeStr=Inherit: Same as input
  Abs : Abs  SaturateOnIntegerOverflow=on
  Math Function : Math  Operator=sqrt  SaturateOnIntegerOverflow=on
  Pipe Section : Gain  Gain=S_p  SaturateOnIntegerOverflow=on  OutDataTypeStr=Inherit: Same as input  ParamDataTypeStr=Inherit: Same as input
  Product : Product  SaturateOnIntegerOverflow=on  InputSameDT=on  OutDataTypeStr=Inherit: Same as first input
  Sign : Signum
  Sum : Sum  Inputs=+-  SaturateOnIntegerOverflow=on  InputSameDT=on  OutDataTypeStr=Inherit: Same as first input
  outflow coeff. : Gain  Gain=c_o  SaturateOnIntegerOverflow=on  OutDataTypeStr=Inherit: Same as input  ParamDataTypeStr=Inherit: Same as input
  Outflow : Outport
  wires:
  outflow coeff./1 -> Outflow/1
  Pipe Section/1 -> outflow coeff./1
  Product/1 -> Pipe Section/1
  Sign/1 -> Product/1
  Math Function/1 -> Product/2
  2g/1 -> Math Function/1
  Abs/1 -> 2g/1
  Sum/1 -> Abs/1, Sign/1
  Level 2/1 -> Sum/2
  Level 1/1 -> Sum/1

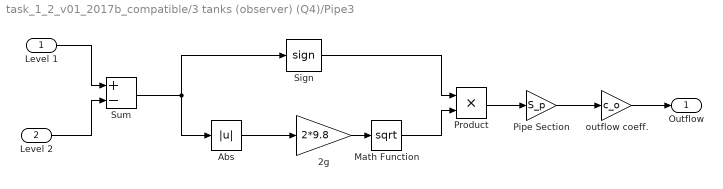
== system task_1_2_v01_2017b_compatible/3 tanks (observer) (Q4)/Pipe3 ==
  Level 1 : Inport
  Level 2 : Inport  Port=2
  2g : Gain  Gain=2*9.8  SaturateOnIntegerOverflow=on  OutDataTypeStr=Inherit: Same as input  ParamDataTypeStr=Inherit: Same as input
  Abs : Abs  SaturateOnIntegerOverflow=on
  Math Function : Math  Operator=sqrt  SaturateOnIntegerOverflow=on
  Pipe Section : Gain  Gain=S_p  SaturateOnIntegerOverflow=on  OutDataTypeStr=Inherit: Same as input  ParamDataTypeStr=Inherit: Same as input
  Product : Product  SaturateOnIntegerOverflow=on  InputSameDT=on  OutDataTypeStr=Inherit: Same as first input
  Sign : Signum
  Sum : Sum  Inputs=+-  SaturateOnIntegerOverflow=on  InputSameDT=on  OutDataTypeStr=Inherit: Same as first input
  outflow coeff. : Gain  Gain=c_o  SaturateOnIntegerOverflow=on  OutDataTypeStr=Inherit: Same as input  ParamDataTypeStr=Inherit: Same as input
  Outflow : Outport
  wires:
  outflow coeff./1 -> Outflow/1
  Pipe Section/1 -> outflow coeff./1
  Product/1 -> Pipe Section/1
  Sign/1 -> Product/1
  Math Function/1 -> Product/2
  2g/1 -> Math Function/1
  Abs/1 -> 2g/1
  Sum/1 -> Abs/1, Sign/1
  Level 2/1 -> Sum/2
  Level 1/1 -> Sum/1

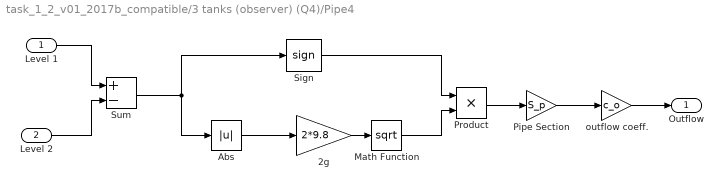
== system task_1_2_v01_2017b_compatible/3 tanks (observer) (Q4)/Pipe4 ==
  Level 1 : Inport
  Level 2 : Inport  Port=2
  2g : Gain  Gain=2*9.8  SaturateOnIntegerOverflow=on  OutDataTypeStr=Inherit: Same as input  ParamDataTypeStr=Inherit: Same as input
  Abs : Abs  SaturateOnIntegerOverflow=on
  Math Function : Math  Operator=sqrt  SaturateOnIntegerOverflow=on
  Pipe Section : Gain  Gain=S_p  SaturateOnIntegerOverflow=on  OutDataTypeStr=Inherit: Same as input  ParamDataTypeStr=Inherit: Same as input
  Product : Product  SaturateOnIntegerOverflow=on  InputSameDT=on  OutDataTypeStr=Inherit: Same as first input
  Sign : Signum
  Sum : Sum  Inputs=+-  SaturateOnIntegerOverflow=on  InputSameDT=on  OutDataTypeStr=Inherit: Same as first input
  outflow coeff. : Gain  Gain=c_o  SaturateOnIntegerOverflow=on  OutDataTypeStr=Inherit: Same as input  ParamDataTypeStr=Inherit: Same as input
  Outflow : Outport
  wires:
  outflow coeff./1 -> Outflow/1
  Pipe Section/1 -> outflow coeff./1
  Product/1 -> Pipe Section/1
  Sign/1 -> Product/1
  Math Function/1 -> Product/2
  2g/1 -> Math Function/1
  Abs/1 -> 2g/1
  Sum/1 -> Abs/1, Sign/1
  Level 2/1 -> Sum/2
  Level 1/1 -> Sum/1

== system task_1_2_v01_2017b_compatible/3 tanks (observer) (Q4)/Tank1 ==
  Inflow : Inport
  Discrete-Time Integrator : DiscreteIntegrator  InitialCondition=x_0  SampleTime=-1  OutMin=min_level  OutMax=max_level  ICPrevOutput=DiscIntNeverNeededParam  ICPrevScaledInput=DiscIntNeverNeededParam
  Tank Section : Gain  Gain=1/S  SaturateOnIntegerOverflow=on  OutDataTypeStr=Inherit: Same as input  ParamDataTypeStr=Inherit: Same as input
  Level : Outport  InitialOutput=0
  wires:
  Discrete-Time Integrator/1 -> Level/1
  Tank Section/1 -> Discrete-Time Integrator/1
  Inflow/1 -> Tank Section/1

== system task_1_2_v01_2017b_compatible/3 tanks (observer) (Q4)/Tank2 ==
  Inflow : Inport
  Discrete-Time Integrator : DiscreteIntegrator  InitialCondition=x_0  SampleTime=-1  OutMin=min_level  OutMax=max_level  ICPrevOutput=DiscIntNeverNeededParam  ICPrevScaledInput=DiscIntNeverNeededParam
  Tank Section : Gain  Gain=1/S  SaturateOnIntegerOverflow=on  OutDataTypeStr=Inherit: Same as input  ParamDataTypeStr=Inherit: Same as input
  Level : Outport  InitialOutput=0
  wires:
  Inflow/1 -> Tank Section/1
  Discrete-Time Integrator/1 -> Level/1
  Tank Section/1 -> Discrete-Time Integrator/1

== system task_1_2_v01_2017b_compatible/3 tanks (observer) (Q4)/Tank3 ==
  Inflow : Inport
  Discrete-Time Integrator : DiscreteIntegrator  InitialCondition=x_0  SampleTime=-1  OutMin=min_level  OutMax=max_level  ICPrevOutput=DiscIntNeverNeededParam  ICPrevScaledInput=DiscIntNeverNeededParam
  Tank Section : Gain  Gain=1/S  SaturateOnIntegerOverflow=on  OutDataTypeStr=Inherit: Same as input  ParamDataTypeStr=Inherit: Same as input
  Level : Outport  InitialOutput=0
  wires:
  Discrete-Time Integrator/1 -> Level/1
  Inflow/1 -> Tank Section/1
  Tank Section/1 -> Discrete-Time Integrator/1

== system task_1_2_v01_2017b_compatible/3 tanks (observer) (Q4)/Valve ==
  In1 : Inport
  Enable : EnablePort  StatesWhenEnabling=reset  ShowOutputPort=on
  Product : Product  SaturateOnIntegerOverflow=on  InputSameDT=on  OutDataTypeStr=Inherit: Same as first input
  Saturation : Saturate  UpperLimit=1.0  LowerLimit=0.0
  Out1 : Outport  OutputWhenDisabled=reset  InitialOutput=0
  wires:
  Enable/1 -> Saturation/1
  Saturation/1 -> Product/1
  In1/1 -> Product/2
  Product/1 -> Out1/1

== system task_1_2_v01_2017b_compatible/3 tanks (observer) (Q4)/Valve1 ==
  In1 : Inport
  Enable : EnablePort  StatesWhenEnabling=reset  ShowOutputPort=on
  Product : Product  SaturateOnIntegerOverflow=on  InputSameDT=on  OutDataTypeStr=Inherit: Same as first input
  Saturation : Saturate  UpperLimit=1.0  LowerLimit=0.0
  Out1 : Outport  OutputWhenDisabled=reset  InitialOutput=0
  wires:
  Enable/1 -> Saturation/1
  Saturation/1 -> Product/1
  In1/1 -> Product/2
  Product/1 -> Out1/1

== system task_1_2_v01_2017b_compatible/3 tanks (observer) (Q4)/Valve2 ==
  In1 : Inport
  Enable : EnablePort  StatesWhenEnabling=reset  ShowOutputPort=on
  Product : Product  SaturateOnIntegerOverflow=on  InputSameDT=on  OutDataTypeStr=Inherit: Same as first input
  Saturation : Saturate  UpperLimit=1.0  LowerLimit=0.0
  Out1 : Outport  OutputWhenDisabled=reset  InitialOutput=0
  wires:
  Enable/1 -> Saturation/1
  Saturation/1 -> Product/1
  In1/1 -> Product/2
  Product/1 -> Out1/1

== system task_1_2_v01_2017b_compatible/3 tanks (real)/Pipe1 ==
  Level 1 : Inport
  Level 2 : Inport  Port=2
  2g : Gain  Gain=2*9.8  SaturateOnIntegerOverflow=on  OutDataTypeStr=Inherit: Same as input  ParamDataTypeStr=Inherit: Same as input
  Abs : Abs  SaturateOnIntegerOverflow=on
  Math Function : Math  Operator=sqrt  SaturateOnIntegerOverflow=on
  Pipe Section : Gain  Gain=S_p  SaturateOnIntegerOverflow=on  OutDataTypeStr=Inherit: Same as input  ParamDataTypeStr=Inherit: Same as input
  Product : Product  SaturateOnIntegerOverflow=on  InputSameDT=on  OutDataTypeStr=Inherit: Same as first input
  Sign : Signum
  Sum : Sum  Inputs=+-  SaturateOnIntegerOverflow=on  InputSameDT=on  OutDataTypeStr=Inherit: Same as first input
  outflow coeff. : Gain  Gain=c_o  SaturateOnIntegerOverflow=on  OutDataTypeStr=Inherit: Same as input  ParamDataTypeStr=Inherit: Same as input
  Outflow : Outport
  wires:
  outflow coeff./1 -> Outflow/1
  Pipe Section/1 -> outflow coeff./1
  Product/1 -> Pipe Section/1
  Sign/1 -> Product/1
  Math Function/1 -> Product/2
  2g/1 -> Math Function/1
  Abs/1 -> 2g/1
  Sum/1 -> Abs/1, Sign/1
  Level 2/1 -> Sum/2
  Level 1/1 -> Sum/1

== system task_1_2_v01_2017b_compatible/3 tanks (real)/Pipe2 ==
  Level 1 : Inport
  Level 2 : Inport  Port=2
  2g : Gain  Gain=2*9.8  SaturateOnIntegerOverflow=on  OutDataTypeStr=Inherit: Same as input  ParamDataTypeStr=Inherit: Same as input
  Abs : Abs  SaturateOnIntegerOverflow=on
  Math Function : Math  Operator=sqrt  SaturateOnIntegerOverflow=on
  Pipe Section : Gain  Gain=S_p  SaturateOnIntegerOverflow=on  OutDataTypeStr=Inherit: Same as input  ParamDataTypeStr=Inherit: Same as input
  Product : Product  SaturateOnIntegerOverflow=on  InputSameDT=on  OutDataTypeStr=Inherit: Same as first input
  Sign : Signum
  Sum : Sum  Inputs=+-  SaturateOnIntegerOverflow=on  InputSameDT=on  OutDataTypeStr=Inherit: Same as first input
  outflow coeff. : Gain  Gain=c_o  SaturateOnIntegerOverflow=on  OutDataTypeStr=Inherit: Same as input  ParamDataTypeStr=Inherit: Same as input
  Outflow : Outport
  wires:
  outflow coeff./1 -> Outflow/1
  Pipe Section/1 -> outflow coeff./1
  Product/1 -> Pipe Section/1
  Sign/1 -> Product/1
  Math Function/1 -> Product/2
  2g/1 -> Math Function/1
  Abs/1 -> 2g/1
  Sum/1 -> Abs/1, Sign/1
  Level 2/1 -> Sum/2
  Level 1/1 -> Sum/1

== system task_1_2_v01_2017b_compatible/3 tanks (real)/Pipe3 ==
  Level 1 : Inport
  Level 2 : Inport  Port=2
  2g : Gain  Gain=2*9.8  SaturateOnIntegerOverflow=on  OutDataTypeStr=Inherit: Same as input  ParamDataTypeStr=Inherit: Same as input
  Abs : Abs  SaturateOnIntegerOverflow=on
  Math Function : Math  Operator=sqrt  SaturateOnIntegerOverflow=on
  Pipe Section : Gain  Gain=S_p  SaturateOnIntegerOverflow=on  OutDataTypeStr=Inherit: Same as input  ParamDataTypeStr=Inherit: Same as input
  Product : Product  SaturateOnIntegerOverflow=on  InputSameDT=on  OutDataTypeStr=Inherit: Same as first input
  Sign : Signum
  Sum : Sum  Inputs=+-  SaturateOnIntegerOverflow=on  InputSameDT=on  OutDataTypeStr=Inherit: Same as first input
  outflow coeff. : Gain  Gain=c_o  SaturateOnIntegerOverflow=on  OutDataTypeStr=Inherit: Same as input  ParamDataTypeStr=Inherit: Same as input
  Outflow : Outport
  wires:
  outflow coeff./1 -> Outflow/1
  Pipe Section/1 -> outflow coeff./1
  Product/1 -> Pipe Section/1
  Sign/1 -> Product/1
  Math Function/1 -> Product/2
  2g/1 -> Math Function/1
  Abs/1 -> 2g/1
  Sum/1 -> Abs/1, Sign/1
  Level 2/1 -> Sum/2
  Level 1/1 -> Sum/1

== system task_1_2_v01_2017b_compatible/3 tanks (real)/Pipe4 ==
  Level 1 : Inport
  Level 2 : Inport  Port=2
  2g : Gain  Gain=2*9.8  SaturateOnIntegerOverflow=on  OutDataTypeStr=Inherit: Same as input  ParamDataTypeStr=Inherit: Same as input
  Abs : Abs  SaturateOnIntegerOverflow=on
  Math Function : Math  Operator=sqrt  SaturateOnIntegerOverflow=on
  Pipe Section : Gain  Gain=S_p  SaturateOnIntegerOverflow=on  OutDataTypeStr=Inherit: Same as input  ParamDataTypeStr=Inherit: Same as input
  Product : Product  SaturateOnIntegerOverflow=on  InputSameDT=on  OutDataTypeStr=Inherit: Same as first input
  Sign : Signum
  Sum : Sum  Inputs=+-  SaturateOnIntegerOverflow=on  InputSameDT=on  OutDataTypeStr=Inherit: Same as first input
  outflow coeff. : Gain  Gain=c_o  SaturateOnIntegerOverflow=on  OutDataTypeStr=Inherit: Same as input  ParamDataTypeStr=Inherit: Same as input
  Outflow : Outport
  wires:
  outflow coeff./1 -> Outflow/1
  Pipe Section/1 -> outflow coeff./1
  Product/1 -> Pipe Section/1
  Sign/1 -> Product/1
  Math Function/1 -> Product/2
  2g/1 -> Math Function/1
  Abs/1 -> 2g/1
  Sum/1 -> Abs/1, Sign/1
  Level 2/1 -> Sum/2
  Level 1/1 -> Sum/1

== system task_1_2_v01_2017b_compatible/3 tanks (real)/Tank1 ==
  Inflow : Inport
  Initial Level : Constant  Value=x_0
  Integrator : Integrator  InitialConditionSource=external  LimitOutput=on  UpperSaturationLimit=max_level  LowerSaturationLimit=min_level
  Tank Section : Gain  Gain=1/S  SaturateOnIntegerOverflow=on  OutDataTypeStr=Inherit: Same as input  ParamDataTypeStr=Inherit: Same as input
  Level : Outport  InitialOutput=0
  wires:
  Integrator/1 -> Level/1
  Initial Level/1 -> Integrator/2
  Tank Section/1 -> Integrator/1
  Inflow/1 -> Tank Section/1
